simulink model "PythonBox"  (R2018b)
settings: Solver=VariableStepAuto  StartTime=0.0  StopTime=inf  FixedStep=3  RelTol=1e-3
undefined symbols (not defined in the file or in its folder): currentCFG_PythonBox_UR, UR
libraries: gtecHighspeedLib x1, gUSBamplib x1
settings Model: Creator=Tengbuk  LastModifiedBy=User

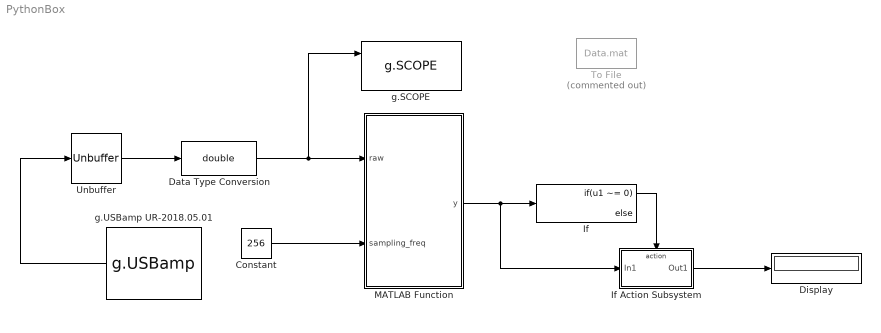
== system PythonBox ==
  Constant : Constant  Value=256
  Data Type Conversion : DataTypeConversion  OutDataTypeStr=double
  Display : Display
  If : If  IfExpression=u1 ~= 0
  If Action Subsystem : Subsystem  TreatAsAtomicUnit=on
  MATLAB Function : MATLAB Function  TreatAsAtomicUnit=on
  To File : ToFile  Commented=on  Filename=Data.mat  SaveFormat=Timeseries
  Unbuffer : Unbuffer
  g.SCOPE : gtecHighspeedLib/g.SCOPE
      settings: SourceProductName=g.tec Highspeed Library
  g.USBamp UR-2018.05.01 : gUSBamplib/g.USBamp  cfg=currentCFG_PythonBox_UR-2018.05.01.cfg  snr=UR-2018.05.01
      settings: SourceProductName=g.USBamp
  wires:
  g.USBamp UR-2018.05.01/1 -> Unbuffer/1
  Unbuffer/1 -> Data Type Conversion/1
  MATLAB Function/1(y) -> If Action Subsystem/1(In1), If/1
  If/1 -> If Action Subsystem/Action
  If Action Subsystem/1(Out1) -> Display/1
  Constant/1 -> MATLAB Function/2(sampling_freq)
  Data Type Conversion/1 -> MATLAB Function/1(raw), g.SCOPE/1

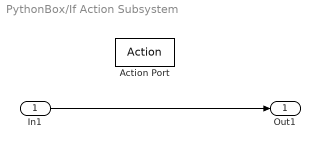
== system PythonBox/If Action Subsystem ==
  In1 : Inport
  Action Port : ActionPort  InitializeStates=reset  ActionType=then
  Out1 : Outport
  wires:
  In1/1 -> Out1/1

== matlab function PythonBox/MATLAB Function ==
  data: raw input; y output; sampling_freq input
function y = pyBlock(raw, sampling_freq)
coder.extrinsic('py.Frequency_recognition_function.fbcca')
coder.extrinsic('py.numpy.ndarray')

% Assign the type of output y
y = 0; 

raw = py.numpy.ndarray(raw, py.numpy.dtype('float64'));

% Run the function in python
output = py.Frequency_recognition_function.fbcca(raw,  sampling_freq);

y = output;
